simulink model "Three_Phase_Rectifier"  (R2020a)
settings: Solver=VariableStepAuto  StartTime=0.0  StopTime=30  RelTol=1e-3
libraries: powerlib x15
settings Model: Creator=Kritika  LastModifiedBy=Kritika

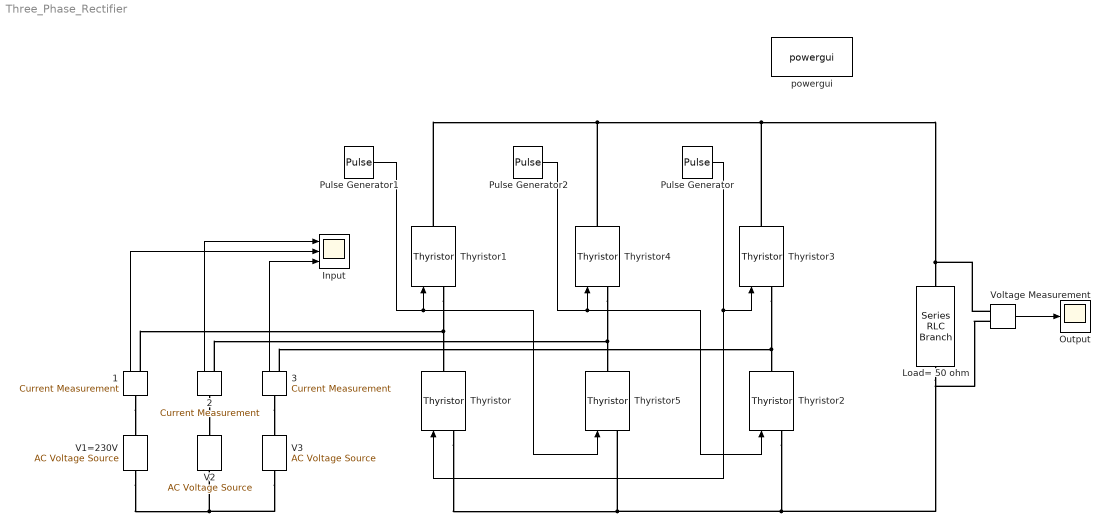
== system Three_Phase_Rectifier ==
  1 : powerlib/Measurements/Current Measurement  PhasorSimulation=off  OutputType=Complex  PSBequivalent=0
  2 : powerlib/Measurements/Current Measurement  PhasorSimulation=off  OutputType=Complex  PSBequivalent=0
  3 : powerlib/Measurements/Current Measurement  PhasorSimulation=off  OutputType=Complex  PSBequivalent=0
  Input : Scope  NumInputPorts=3
  Load= 50 ohm : powerlib/Elements/Series RLC Branch  LConnTagsString=__new0  RConnTagsString=__new0  BranchType=R  Resistance=50  Inductance=1e-3  SetiL0=off  InitialCurrent=0  Capacitance=1e-6  Setx0=off  InitialVoltage=0  Measurements=None
  Output : Scope
  Pulse Generator : DiscretePulseGenerator  PulseType=Time based  Amplitude=10  Period=0.02  PulseWidth=50  PhaseDelay=0.02*(270/360)
  Pulse Generator1 : DiscretePulseGenerator  PulseType=Time based  Amplitude=10  Period=.02  PulseWidth=50  PhaseDelay=0.02*(30/360)
  Pulse Generator2 : DiscretePulseGenerator  PulseType=Time based  Amplitude=10  Period=0.02  PulseWidth=50  PhaseDelay=0.02*(150/360)
  Thyristor{,1..5} (6 alike) : powerlib/Power Electronics/Thyristor  Ron=0.001  Lon=0  Vf=0.8  IC=0  Rs=500  Cs=250e-9  Measurements=off
  V1=230V : powerlib/Electrical Sources/AC Voltage Source  Amplitude=230  Phase=0  Frequency=50  SampleTime=0  Measurements=None  BusType=swing  Pref=10e3  Qref=0  Qmin=-inf  Qmax=+inf
  V2 : powerlib/Electrical Sources/AC Voltage Source  Amplitude=230  Phase=-120  Frequency=50  SampleTime=0  Measurements=None  BusType=swing  Pref=10e3  Qref=0  Qmin=-inf  Qmax=+inf
  V3 : powerlib/Electrical Sources/AC Voltage Source  Amplitude=230  Phase=120  Frequency=50  SampleTime=0  Measurements=None  BusType=swing  Pref=10e3  Qref=0  Qmin=-inf  Qmax=+inf
  Voltage Measurement : powerlib/Measurements/Voltage Measurement  PhasorSimulation=off  OutputType=Complex  PSBequivalent=0
  powergui : powerlib/powergui  Priority=1  SimulationMode=Continuous  SampleTime=50e-6  frequency=60  Iterations=50  frequencyindice=50  Pbase=100e6  ErrMax=1e-4  UnitsV=kV  UnitsW=MW  buscounter=0  FunctionMessages=off  echomessages=off  EnableUseOfTLC=off  CurrentSourceSwitches=off  DisableSnubberDevices=off  DisableRonSwitches=off  DisableVfSwitches=off  DisplayEquations=off  AutomaticDiscreteSolvers=off  SolverType=Tustin/Backward Euler (TBE)  Interpol=off  ExternalGateDelay=off  methode=off  Ts=100  x0status=blocks  SPID=on  SwTol=0  HookPort=off  NonlinearTolerance=1e-4  nMaxIteration=100  ContinueOnMaxIteration=off  RestoreLinks=warning  ResistiveCurrentMeasurement=off  Frange=[0:2:500]  Ylog=off  Xlog=on  ShowGrid=off  save=off  variable=ZData  structure=0  ZoomFFT=off  StartTime=0.0  cycles=1  DisplayStyle=1  fundamental=60  FreqAxis=off  MaxFrequency=1000  frequencyindicesteady=1  RmsSteady=1  display=off
  wires:
  Pulse Generator1/1 -> Thyristor5/1, Thyristor1/1
  Pulse Generator2/1 -> Thyristor2/1, Thyristor4/1
  Pulse Generator/1 -> Thyristor3/1, Thyristor/1
  Voltage Measurement/1 -> Output/1
  1/1 -> Input/2
  2/1 -> Input/1
  3/1 -> Input/3
  connections:
  Thyristor1/RConn1 -- Voltage Measurement/LConn1 -- Load= 50 ohm/LConn1 -- Thyristor3/RConn1 -- Thyristor4/RConn1
  Thyristor1/LConn1 -- 1/RConn1 -- Thyristor/RConn1
  Thyristor4/LConn1 -- 2/RConn1 -- Thyristor5/RConn1
  Thyristor3/LConn1 -- 3/RConn1 -- Thyristor2/RConn1
  V1=230V/LConn1 -- V2/LConn1 -- V3/LConn1
  Thyristor/LConn1 -- Load= 50 ohm/RConn1 -- Voltage Measurement/LConn2 -- Thyristor2/LConn1 -- Thyristor5/LConn1
  1/LConn1 -- V1=230V/RConn1
  2/LConn1 -- V2/RConn1
  3/LConn1 -- V3/RConn1
